simulink model "x_Part_11_Modern_Controller"  (R2025b)
settings: Solver=VariableStepAuto  StartTime=0.0  StopTime=10.0  RelTol=1e-3
values from neighbouring files (symbols this model uses):
  A = [0,             1,            0,                0 ... (first row only)    [Part11_Modern_Controller_ELEC481.m]    (also in Part9_10_Modern_Controller_ELEC481.m; sys_params.m = [0,        1,         0,        0)
  A_obs = A - L*C    [Part11_Modern_Controller_ELEC481.m]    (also in Part9_10_Modern_Controller_ELEC481.m)
  B = [0 ... (first row only)    [Part11_Modern_Controller_ELEC481.m]    (also in Part9_10_Modern_Controller_ELEC481.m; sys_params.m = [0; khw/J1; 0; 0])
  B_obs = [B, L]    [Part11_Modern_Controller_ELEC481.m]    (also in Part9_10_Modern_Controller_ELEC481.m)
  C = [1, 0, 0, 0 ... (first row only)    [Part11_Modern_Controller_ELEC481.m]    (also in Part9_10_Modern_Controller_ELEC481.m; sys_params.m)
  C_obs = eye(4)    [Part11_Modern_Controller_ELEC481.m]    (also in Part9_10_Modern_Controller_ELEC481.m = eye(size(A)))
  D = [0 ... (first row only)    [Part11_Modern_Controller_ELEC481.m]    (also in Part9_10_Modern_Controller_ELEC481.m; sys_params.m = [0; 0])
  D_obs = zeros(4, 3)    [Part11_Modern_Controller_ELEC481.m]    (also in Part9_10_Modern_Controller_ELEC481.m = [zeros(size(B)), zeros(size(L))])
  K = place(A, B, P_controller)    [Part11_Modern_Controller_ELEC481.m]    (also in Part9_10_Modern_Controller_ELEC481.m)
  Nbar = 1 / gain    [Part11_Modern_Controller_ELEC481.m]    (also in Part9_10_Modern_Controller_ELEC481.m)

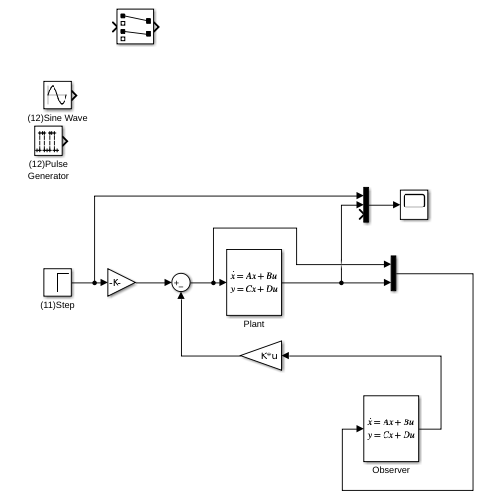
[thumbnail: Simulink's stored preview of the top-level diagram]
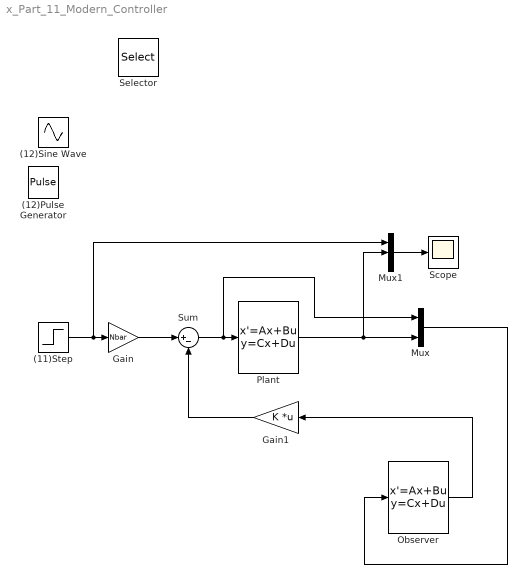
== system x_Part_11_Modern_Controller ==
  (11)Step : Step  SampleTime=0
  (12)Pulse Generator : DiscretePulseGenerator  Period=4  PulseWidth=2
  (12)Sine Wave : Sin  SampleTime=0
  Gain : Gain  Gain=Nbar
  Gain1 : Gain  Gain=K  Multiplication=Matrix(K*u)
  Mux : Mux  Inputs=2
  Mux1 : Mux  Inputs=3
  Observer : StateSpace  A=A_obs  B=B_obs  C=C_obs  D=D_obs  InitialCondition=[0; 0; 0; 0]
  Plant : StateSpace  A=A  B=B  C=C  D=D  InitialCondition=[0.1; 0; 0; 0]
  Scope : Scope
      settings: ActiveDisplayYMinimum=-0.18890066790016624  ActiveDisplayYMaximum=1.9995628826792948
  Selector : Selector  InputPortWidth=4  IndexOptions=Index vector (dialog)  Indices=[1 3]  OutputSizes=1
  Sum : Sum  Inputs=|+-
  wires:
  (11)Step/1 -> Mux1/1, Gain/1
  Gain/1 -> Sum/1
  Gain1/1 -> Sum/2
  Observer/1 -> Gain1/1
  Sum/1 -> Mux/1, Plant/1
  Plant/1 -> Mux1/2, Mux/2
  Mux/1 -> Observer/1
  Mux1/1 -> Scope/1
